simulink model "RealAndSimulatedPlantBlock2019"  (R2019b)
settings: Solver=FixedStepAuto  StartTime=0.0  StopTime=60  FixedStep=0.001  RelTol=1e-3
values from neighbouring files (symbols this model uses):
  A = [0 0 0 0 1 -7.46314951586 0 9.2203186001 0 -3.6743536316 0 36.5167723042 ... (16 elements, 4x4)]    [PlantParams.mat]
  B = [0 5.59662878796 0 -6.91433293703]    [PlantParams.mat]
  c = 0.2    [PlantParams.mat]    (also in params.m = 0.1)
  dtheta1 = 41.8879020479    [PlantParams.mat]    (also in params.m)
  g = 9.81    [PlantParams.mat]    (also in params.m)
  Id = 0.0148    [PlantParams.mat]    (also in params.m)
  ID = 0.0148142940058    [PlantParams.mat]
  J1 = 0.13138281053    [PlantParams.mat]    (also in params.m = 0.1314)
  JC = 0.0268600431258    [PlantParams.mat]
  JD = 0.0273039035837    [PlantParams.mat]
  Jz_bar = 0.0130765    [PlantParams.mat]    (also in params.m = 0.0131)
  lcg = 0.269778481013    [PlantParams.mat]    (also in params.m = 0.2698)
  m = 0.158    [PlantParams.mat]    (also in params.m)
  rh = 0.37    [PlantParams.mat]    (also in params.m)
undefined symbols (not defined in the file or in its folder): C, D, X, Y, Z
libraries: sm_lib x20, nesl_utility x5, simulink x1
(part 1 of 2)
settings Model: EnablePacing=on  Creator=samue  LastModifiedBy=samue
settings DebuggingCC: SFMachineParentedDataDiag=error

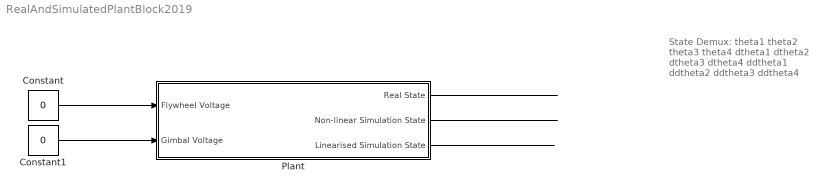
== system RealAndSimulatedPlantBlock2019 ==
  note: State Demux:
      | theta1
      | theta2
      | theta3
      | theta4
      | dtheta1
      | dtheta2
      | dtheta3
      | dtheta4
      | ddtheta1
      | ddtheta2
      | ddtheta3
      | ddtheta4
  Constant : Constant  Value=0
  Constant1 : Constant  Value=0
  Plant : Subsystem
  wires:
  Constant/1 -> Plant/1(Flywheel Voltage)
  Constant1/1 -> Plant/2(Gimbal Voltage)
  Plant/1(Real State) -> ?
  Plant/2(Non-linear Simulation State) -> ?
  Plant/3(Linearised Simulation State) -> ?

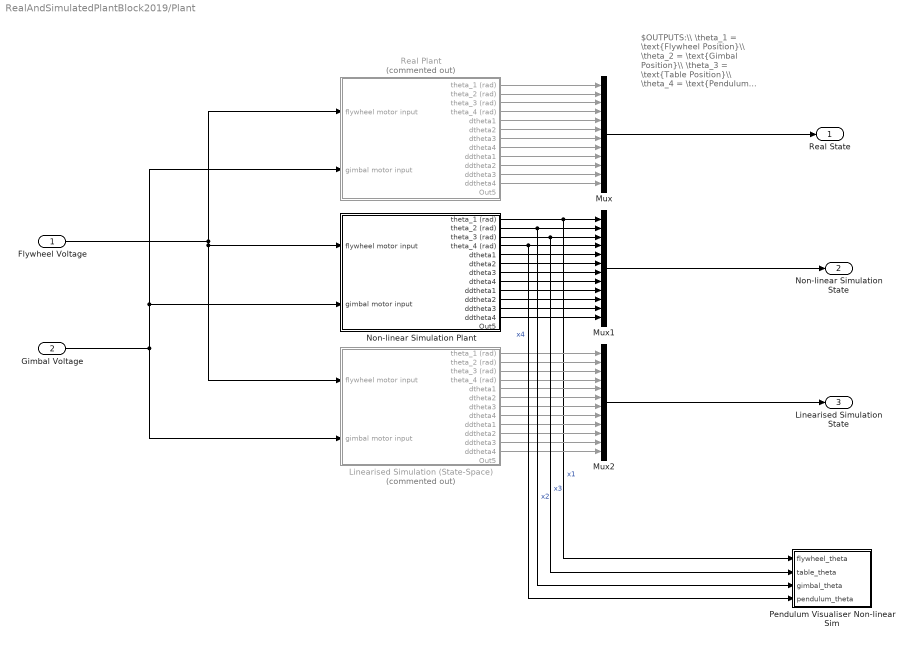
== system RealAndSimulatedPlantBlock2019/Plant ==
  note: $OUTPUTS:\\ \theta_1 = \text{Flywheel Position}\\ \theta_2 = \text{Gimbal Position}\\ \theta_3 = \text{Table Position}\\ \theta_4 = \text{Pendulum Position}\\$
  Flywheel Voltage : Inport
  Gimbal Voltage : Inport  Port=2
  Linearised Simulation (State-Space) : Subsystem  Commented=on
  Mux : Mux  Inputs=12
  Mux1 : Mux  Inputs=12
  Mux2 : Mux  Inputs=12
  Non-linear Simulation Plant : Subsystem
  Pendulum Visualiser Non-linear Sim : Subsystem
  Real Plant : Subsystem  Commented=on
  Real State : Outport
  Non-linear Simulation State : Outport  Port=2
  Linearised Simulation State : Outport  Port=3
  wires:
  Gimbal Voltage/1 -> Linearised Simulation (State-Space)/2(gimbal motor input), Real Plant/2(gimbal motor input), Non-linear Simulation Plant/2(gimbal motor input)
  Flywheel Voltage/1 -> Linearised Simulation (State-Space)/1(flywheel motor input), Non-linear Simulation Plant/1(flywheel motor input), Real Plant/1(flywheel motor input)
  Real Plant/3(theta_3 (rad)) -> Mux/3
  Real Plant/1(theta_1 (rad)) -> Mux/1
  Real Plant/4(theta_4 (rad)) -> Mux/4
  Real Plant/2(theta_2 (rad)) -> Mux/2
  Real Plant/5(dtheta1) -> Mux/5
  Real Plant/6(dtheta2) -> Mux/6
  Real Plant/7(dtheta3) -> Mux/7
  Real Plant/8(dtheta4) -> Mux/8
  Real Plant/9(ddtheta1) -> Mux/9
  Real Plant/10(ddtheta2) -> Mux/10
  Real Plant/11(ddtheta3) -> Mux/11
  Real Plant/12(ddtheta4) -> Mux/12
  Mux/1 -> Real State/1
  Non-linear Simulation Plant/9(ddtheta1) -> Mux1/9
  Non-linear Simulation Plant/12(ddtheta4) -> Mux1/12
  Non-linear Simulation Plant/1(theta_1 (rad)) -> Pendulum Visualiser Non-linear Sim/1(flywheel_theta), Mux1/1  "x1"
  Non-linear Simulation Plant/7(dtheta3) -> Mux1/7
  Non-linear Simulation Plant/10(ddtheta2) -> Mux1/10
  Non-linear Simulation Plant/11(ddtheta3) -> Mux1/11
  Non-linear Simulation Plant/8(dtheta4) -> Mux1/8
  Non-linear Simulation Plant/6(dtheta2) -> Mux1/6
  Non-linear Simulation Plant/5(dtheta1) -> Mux1/5
  Mux1/1 -> Non-linear Simulation State/1
  Linearised Simulation (State-Space)/3(theta_3 (rad)) -> Mux2/3
  Linearised Simulation (State-Space)/9(ddtheta1) -> Mux2/9
  Linearised Simulation (State-Space)/4(theta_4 (rad)) -> Mux2/4
  Linearised Simulation (State-Space)/7(dtheta3) -> Mux2/7
  Linearised Simulation (State-Space)/5(dtheta1) -> Mux2/5
  Linearised Simulation (State-Space)/12(ddtheta4) -> Mux2/12
  Linearised Simulation (State-Space)/1(theta_1 (rad)) -> Mux2/1
  Linearised Simulation (State-Space)/10(ddtheta2) -> Mux2/10
  Linearised Simulation (State-Space)/11(ddtheta3) -> Mux2/11
  Linearised Simulation (State-Space)/8(dtheta4) -> Mux2/8
  Mux2/1 -> Linearised Simulation State/1
  Linearised Simulation (State-Space)/6(dtheta2) -> Mux2/6
  Linearised Simulation (State-Space)/2(theta_2 (rad)) -> Mux2/2
  Non-linear Simulation Plant/4(theta_4 (rad)) -> Pendulum Visualiser Non-linear Sim/4(pendulum_theta), Mux1/4  "x4"
  Non-linear Simulation Plant/2(theta_2 (rad)) -> Pendulum Visualiser Non-linear Sim/3(gimbal_theta), Mux1/2  "x2"
  Non-linear Simulation Plant/3(theta_3 (rad)) -> Pendulum Visualiser Non-linear Sim/2(table_theta), Mux1/3  "x3"

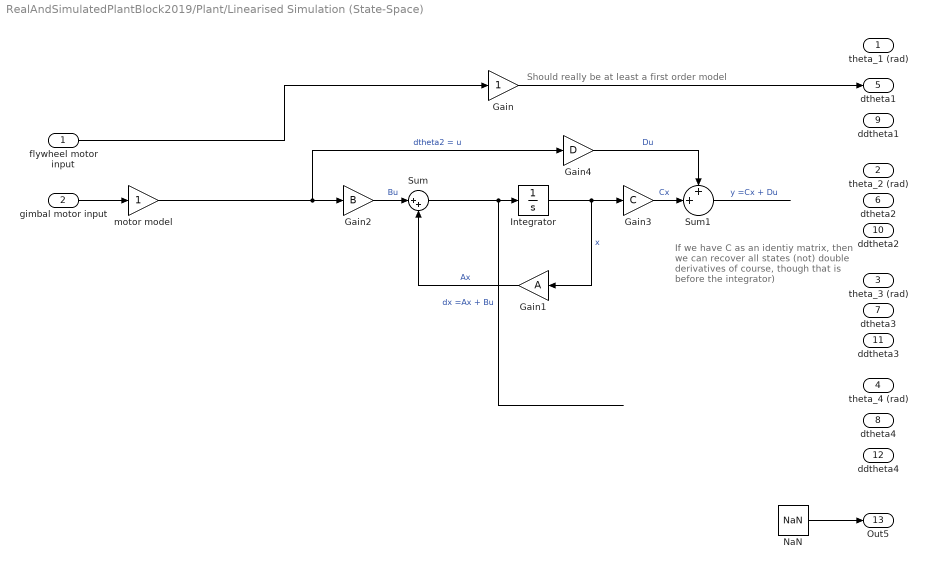
== system RealAndSimulatedPlantBlock2019/Plant/Linearised Simulation (State-Space) ==
  note: If we have C as an identiy matrix,
      | then we can recover all states (not)
      | double derivatives of course, though
      | that is before the integrator)
  note: Should really be at least a first order model
  flywheel motor input : Inport
  gimbal motor input : Inport  Port=2
  Gain : Gain
  Gain1 : Gain  Gain=A
  Gain2 : Gain  Gain=B
  Gain3 : Gain  Gain=C
  Gain4 : Gain  Gain=D
  Integrator : Integrator
  NaN : Constant  Value=NaN  OutDataTypeStr=Inherit: Inherit via back propagation
  Sum : Sum  Inputs=|++
  Sum1 : Sum  Inputs=++|
  motor model : Gain
  theta_1 (rad) : Outport
  theta_2 (rad) : Outport  Port=2
  theta_3 (rad) : Outport  Port=3
  theta_4 (rad) : Outport  Port=4
  dtheta1 : Outport  Port=5
  dtheta2 : Outport  Port=6
  dtheta3 : Outport  Port=7
  dtheta4 : Outport  Port=8
  ddtheta1 : Outport  Port=9
  ddtheta2 : Outport  Port=10
  ddtheta3 : Outport  Port=11
  ddtheta4 : Outport  Port=12
  Out5 : Outport  Port=13
  wires:
  gimbal motor input/1 -> motor model/1
  NaN/1 -> Out5/1
  flywheel motor input/1 -> Gain/1
  Gain/1 -> dtheta1/1
  Integrator/1 -> Gain3/1, Gain1/1  "x"
  Gain1/1 -> Sum/2  "Ax"
  Sum/1 -> Integrator/1  "dx =Ax + Bu"
  Gain2/1 -> Sum/1  "Bu"
  motor model/1 -> Gain2/1, Gain4/1  "dtheta2 = u"
  Gain3/1 -> Sum1/2  "Cx"
  Gain4/1 -> Sum1/1  "Du"
  Sum1/1 -> ?  "y =Cx + Du"

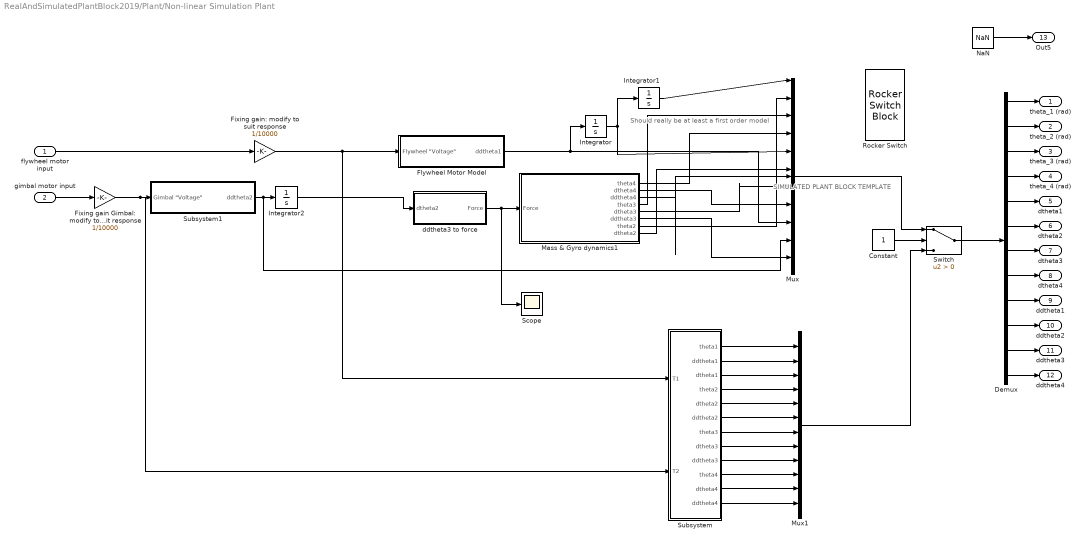
== system RealAndSimulatedPlantBlock2019/Plant/Non-linear Simulation Plant ==
  note: SIMULATED PLANT BLOCK TEMPLATE
  note: Should really be at least a first order model
  flywheel motor input : Inport
  gimbal motor input : Inport  Port=2
  Constant : Constant
  Demux : Demux  Outputs=12
  Fixing gain Gimbal: modify to suit response : Gain  Gain=1/10000
  Fixing gain: modify to suit response : Gain  Gain=1/10000
  "Flywheel Motor Model " : Subsystem
  Integrator : Integrator
  Integrator1 : Integrator
  Integrator2 : Integrator
  Mass & Gyro dynamics1 : Subsystem
  Mux : Mux  Inputs=12
  Mux1 : Mux  Inputs=12
  NaN : Constant  Value=NaN  OutDataTypeStr=Inherit: Inherit via back propagation
  Rocker Switch : RockerSwitchBlock
      settings: Values={{'Off', 'On'}, [0 1]}
  Scope : Scope
  Subsystem : Subsystem
  Subsystem1 : Subsystem
  Switch : Switch  Criteria=u2 > Threshold
  ddtheta3 to force : Subsystem
  theta_1 (rad) : Outport
  theta_2 (rad) : Outport  Port=2
  theta_3 (rad) : Outport  Port=3
  theta_4 (rad) : Outport  Port=4
  dtheta1 : Outport  Port=5
  dtheta2 : Outport  Port=6
  dtheta3 : Outport  Port=7
  dtheta4 : Outport  Port=8
  ddtheta1 : Outport  Port=9
  ddtheta2 : Outport  Port=10
  ddtheta3 : Outport  Port=11
  ddtheta4 : Outport  Port=12
  Out5 : Outport  Port=13
  wires:
  gimbal motor input/1 -> Fixing gain Gimbal: modify to suit response/1
  NaN/1 -> Out5/1
  Subsystem1/1(ddtheta2) -> Mux/10, Integrator2/1
  Mass & Gyro dynamics1/7(theta2) -> Mux/2
  Mass & Gyro dynamics1/8(dtheta2) -> Mux/6
  Mass & Gyro dynamics1/4(theta3) -> Mux/3
  Mass & Gyro dynamics1/5(dtheta3) -> Mux/7
  Mass & Gyro dynamics1/6(ddtheta3) -> Mux/11
  Mass & Gyro dynamics1/1(theta4) -> Mux/4
  Mass & Gyro dynamics1/2(dtheta4) -> Mux/8
  Mass & Gyro dynamics1/3(ddtheta4) -> Mux/12
  flywheel motor input/1 -> Fixing gain: modify to suit response/1
  ddtheta3 to force/1(Force) -> Scope/1, Mass & Gyro dynamics1/1(Force)
  Integrator2/1 -> ddtheta3 to force/1(dtheta2)
  "Flywheel Motor Model "/1(ddtheta1) -> Mux/9, Integrator/1
  Fixing gain: modify to suit response/1 -> Subsystem/1(T1), "Flywheel Motor Model "/1("Flywheel \"Voltage\"")
  Integrator/1 -> Integrator1/1, Mux/5
  Integrator1/1 -> Mux/1
  Fixing gain Gimbal: modify to suit response/1 -> Subsystem/2(T2), Subsystem1/1("Gimbal \"Voltage\"")
  Subsystem/1(theta1) -> Mux1/1
  Subsystem/2(ddtheta1) -> Mux1/2
  Subsystem/3(dtheta1) -> Mux1/3
  Subsystem/4("theta2 ") -> Mux1/4
  Subsystem/6(ddtheta2) -> Mux1/6
  Subsystem/5(dtheta2) -> Mux1/5
  Subsystem/7(theta3) -> Mux1/7
  Subsystem/8(dtheta3) -> Mux1/8
  Subsystem/9(ddtheta3) -> Mux1/9
  Subsystem/10(theta4) -> Mux1/10
  Subsystem/11(dtheta4) -> Mux1/11
  Subsystem/12("ddtheta4 ") -> Mux1/12
  Demux/1 -> theta_1 (rad)/1
  Demux/2 -> theta_2 (rad)/1
  Demux/3 -> theta_3 (rad)/1
  Demux/4 -> theta_4 (rad)/1
  Demux/5 -> dtheta1/1
  Demux/6 -> dtheta2/1
  Demux/7 -> dtheta3/1
  Demux/8 -> dtheta4/1
  Demux/9 -> ddtheta1/1
  Demux/10 -> ddtheta2/1
  Demux/11 -> ddtheta3/1
  Demux/12 -> ddtheta4/1
  Constant/1 -> Switch/2
  Mux/1 -> Switch/1
  Mux1/1 -> Switch/3
  Switch/1 -> Demux/1

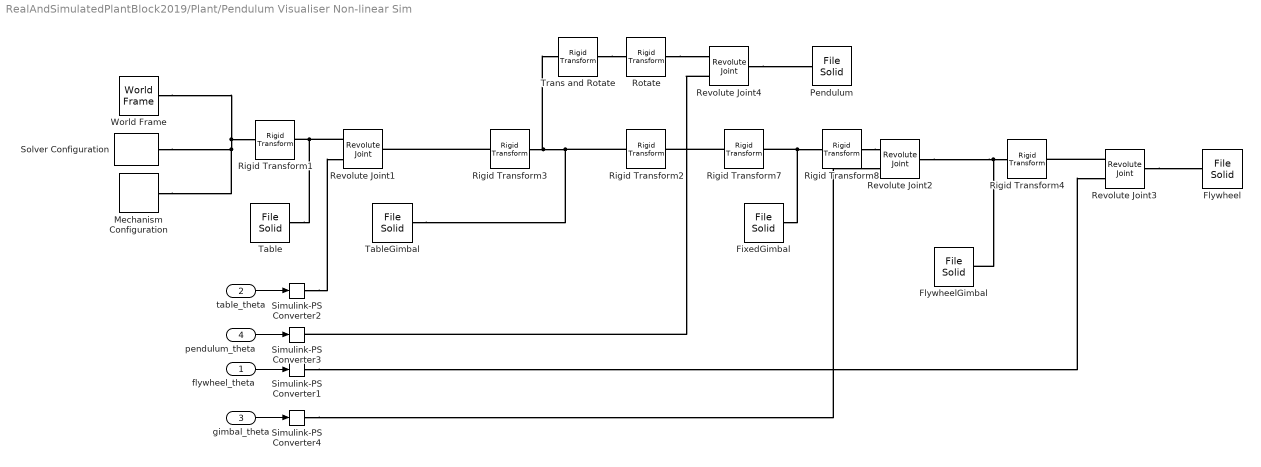
== system RealAndSimulatedPlantBlock2019/Plant/Pendulum Visualiser Non-linear Sim ==
  flywheel_theta : Inport
  table_theta : Inport  Port=2
  gimbal_theta : Inport  Port=3
  pendulum_theta : Inport  Port=4
  FixedGimbal : sm_lib/Body Elements/File Solid  ExtGeomFileName=C:\Users\samue\OneDrive\METR6203\CAD\gimbal_fixed.stp  UnitType=FromFile  ExtGeomFileUnits=m  StepReaderType=HEX  ExportEntireGeometry=off  InertiaType=CalculateFromGeometry  Mass=1  MassUnits=kg  CenterOfMass=[0 0 0]  CenterOfMassUnits=m  MomentsOfInertia=[1 1 1]  MomentsOfInertiaUnits=kg*m^2  ProductsOfInertia=[0 0 0]  ProductsOfInertiaUnits=kg*m^2  BasedOnType=Density  Density=1000  DensityUnits=kg/m^3  DoExposeReferenceFrame=on  SerializedFrames=<Frames/>  GraphicType=FromGeometry  MarkerShape=Sphere  MarkerSize=10  GraphicVisPropType=SimpleVisualProperties  GraphicDiffuseColor=[0.2 0.2 0.2]  GraphicSpecularColor=[0.5 0.5 0.5 1.0]  GraphicAmbientColor=[0.15 0.15 0.15 1.0]  GraphicEmissiveColor=[0.0 0.0 0.0 1.0]  GraphicShininess=75  GraphicOpacity=1.0
  Flywheel : sm_lib/Body Elements/File Solid  ExtGeomFileName=C:\Users\samue\OneDrive\METR6203\CAD\flywheel.stp  UnitType=FromFile  ExtGeomFileUnits=m  StepReaderType=HEX  ExportEntireGeometry=off  InertiaType=CalculateFromGeometry  Mass=1  MassUnits=kg  CenterOfMass=[0 0 0]  CenterOfMassUnits=m  MomentsOfInertia=[1 1 1]  MomentsOfInertiaUnits=kg*m^2  ProductsOfInertia=[0 0 0]  ProductsOfInertiaUnits=kg*m^2  BasedOnType=Density  Density=1000  DensityUnits=kg/m^3  DoExposeReferenceFrame=on  SerializedFrames=<Frames/>  GraphicType=FromGeometry  MarkerShape=Sphere  MarkerSize=10  GraphicVisPropType=SimpleVisualProperties  GraphicDiffuseColor=[0.8 0.6 0.0]  GraphicSpecularColor=[0.5 0.5 0.5 1.0]  GraphicAmbientColor=[0.15 0.15 0.15 1.0]  GraphicEmissiveColor=[0.0 0.0 0.0 1.0]  GraphicShininess=75  GraphicOpacity=1.0
  FlywheelGimbal : sm_lib/Body Elements/File Solid  ExtGeomFileName=C:\Users\samue\OneDrive\METR6203\CAD\flywheel_gimbal.stp  UnitType=FromFile  ExtGeomFileUnits=m  StepReaderType=HEX  ExportEntireGeometry=off  InertiaType=CalculateFromGeometry  Mass=1  MassUnits=kg  CenterOfMass=[0 0 0]  CenterOfMassUnits=m  MomentsOfInertia=[1 1 1]  MomentsOfInertiaUnits=kg*m^2  ProductsOfInertia=[0 0 0]  ProductsOfInertiaUnits=kg*m^2  BasedOnType=Density  Density=1000  DensityUnits=kg/m^3  DoExposeReferenceFrame=on  SerializedFrames=<Frames/>  GraphicType=FromGeometry  MarkerShape=Sphere  MarkerSize=10  GraphicVisPropType=SimpleVisualProperties  GraphicDiffuseColor=[0.5 0.5 0.5]  GraphicSpecularColor=[0.5 0.5 0.5 1.0]  GraphicAmbientColor=[0.15 0.15 0.15 1.0]  GraphicEmissiveColor=[0.0 0.0 0.0 1.0]  GraphicShininess=75  GraphicOpacity=1.0
  Mechanism Configuration : sm_lib/Utilities/Mechanism Configuration  UniformGravity=Constant  GravityVector=[0 0 -9.80665]  GravityUnits=m/s^2  LinearizationDelta=0.001
  Pendulum : sm_lib/Body Elements/File Solid  ExtGeomFileName=C:\Users\samue\OneDrive\METR6203\CAD\pendulum.stp  UnitType=FromFile  ExtGeomFileUnits=m  StepReaderType=HEX  ExportEntireGeometry=off  InertiaType=CalculateFromGeometry  Mass=1  MassUnits=kg  CenterOfMass=[0 0 0]  CenterOfMassUnits=m  MomentsOfInertia=[1 1 1]  MomentsOfInertiaUnits=kg*m^2  ProductsOfInertia=[0 0 0]  ProductsOfInertiaUnits=kg*m^2  BasedOnType=Density  Density=1000  DensityUnits=kg/m^3  DoExposeReferenceFrame=on  SerializedFrames=<Frames/>  GraphicType=FromGeometry  MarkerShape=Sphere  MarkerSize=10  GraphicVisPropType=SimpleVisualProperties  GraphicDiffuseColor=[0.5 0.5 0.5]  GraphicSpecularColor=[0.5 0.5 0.5 1.0]  GraphicAmbientColor=[0.15 0.15 0.15 1.0]  GraphicEmissiveColor=[0.0 0.0 0.0 1.0]  GraphicShininess=75  GraphicOpacity=1.0
  Revolute Joint{1..4} (4 alike) : sm_lib/Joints/Revolute Joint  JointMode=Normal  SenseConstraintForce=off  SenseConstraintForceX=off  SenseConstraintForceY=off  SenseConstraintForceZ=off  SenseConstraintTorque=off  SenseConstraintTorqueX=off  SenseConstraintTorqueY=off  SenseConstraintTorqueZ=off  SenseTotalForce=off  SenseTotalForceX=off  SenseTotalForceY=off  SenseTotalForceZ=off  SenseTotalTorque=off  SenseTotalTorqueX=off  SenseTotalTorqueY=off  SenseTotalTorqueZ=off  CompositeWrenchDir=FollowerOnBase  CompositeWrenchFrame=BaseFrame  EquilibriumPosition=0  EquilibriumPositionUnits=deg  SpringStiffness=0  SpringStiffnessUnits=N*m/deg  DampingCoefficient=0  DampingCoefficientUnits=N*m/(deg/s)  TorqueActuationMode=ComputedTorque  MotionActuationMode=InputMotion  SensePosition=off  SenseVelocity=off  SenseAcceleration=off  SenseTorqueForce=off  SenseLowerLimitTorqueForce=off  SenseUpperLimitTorqueForce=off  LowerLimitSpecify=off  LowerLimitBound=-90  LowerLimitBoundUnits=deg  LowerLimitStiffness=1e4  LowerLimitStiffnessUnits=N*m/deg  LowerLimitDamping=10  LowerLimitDampingUnits=N*m/(deg/s)  LowerLimitTransitionRegionWidth=0.1  LowerLimitTransitionRegionWidthUnits=deg  UpperLimitSpecify=off  UpperLimitBound=90  UpperLimitBoundUnits=deg  UpperLimitStiffness=1e4  UpperLimitStiffnessUnits=N*m/deg  UpperLimitDamping=10  UpperLimitDampingUnits=N*m/(deg/s)  UpperLimitTransitionRegionWidth=0.1  UpperLimitTransitionRegionWidthUnits=deg  PositionTargetSpecify=off  PositionTargetPriority=High  PositionTargetValue=0  PositionTargetValueUnits=deg  VelocityTargetSpecify=off  VelocityTargetPriority=High  VelocityTargetValue=0  VelocityTargetValueUnits=deg/s
  Rigid Transform1 : sm_lib/Frames and Transforms/Rigid Transform  TranslationMethod=None  TranslationStandardOffset=0  TranslationLengthUnit=m  TranslationStandardAxis=+Z  TranslationCartesianOffset=[0 0 0]  TranslationROffset=0  TranslationROffsetUnits=m  TranslationZOffset=0  TranslationZOffsetUnits=m  TranslationThetaOffset=0  TranslationThetaOffsetUnits=deg  RotationMethod=StandardAxis  RotationAngleUnits=deg  RotationStandardAxis=+X  RotationAngle=0  RotationArbitraryAxis=[0 0 1]  FollAlignAxisA=+X  BaseAlignAxisA=+Y  FollAlignAxisB=+Y  BaseAlignAxisB=+Z  RotationSequenceAxes=FollowerAxes  RotationSequence=XYX  RotationSequenceAngles=[0 0 0]  RotationSequenceAnglesUnits=deg  RotationMatrix=[1 0 0; 0 1 0; 0 0 1]
  Rigid Transform2 : sm_lib/Frames and Transforms/Rigid Transform  TranslationMethod=StandardAxis  TranslationStandardOffset=00  TranslationLengthUnit=m  TranslationStandardAxis=+Y  TranslationCartesianOffset=[0 0 0]  TranslationROffset=0  TranslationROffsetUnits=m  TranslationZOffset=0  TranslationZOffsetUnits=m  TranslationThetaOffset=0  TranslationThetaOffsetUnits=deg  RotationMethod=StandardAxis  RotationAngleUnits=deg  RotationStandardAxis=+X  RotationAngle=90  RotationArbitraryAxis=[0 0 1]  FollAlignAxisA=+X  BaseAlignAxisA=+Y  FollAlignAxisB=+Y  BaseAlignAxisB=+Z  RotationSequenceAxes=FollowerAxes  RotationSequence=XYX  RotationSequenceAngles=[0 0 0]  RotationSequenceAnglesUnits=deg  RotationMatrix=[1 0 0; 0 1 0; 0 0 1]
  Rigid Transform3 : sm_lib/Frames and Transforms/Rigid Transform  TranslationMethod=StandardAxis  TranslationStandardOffset=245+7  TranslationLengthUnit=mm  TranslationStandardAxis=+Z  TranslationCartesianOffset=[0 0 0]  TranslationROffset=0  TranslationROffsetUnits=m  TranslationZOffset=0  TranslationZOffsetUnits=m  TranslationThetaOffset=0  TranslationThetaOffsetUnits=deg  RotationMethod=StandardAxis  RotationAngleUnits=deg  RotationStandardAxis=+X  RotationAngle=0  RotationArbitraryAxis=[0 0 1]  FollAlignAxisA=+X  BaseAlignAxisA=+Y  FollAlignAxisB=+Y  BaseAlignAxisB=+Z  RotationSequenceAxes=FollowerAxes  RotationSequence=XYX  RotationSequenceAngles=[0 0 0]  RotationSequenceAnglesUnits=deg  RotationMatrix=[1 0 0; 0 1 0; 0 0 1]
  Rigid Transform4 : sm_lib/Frames and Transforms/Rigid Transform  TranslationMethod=StandardAxis  TranslationStandardOffset=00  TranslationLengthUnit=m  TranslationStandardAxis=+Y  TranslationCartesianOffset=[0 0 0]  TranslationROffset=0  TranslationROffsetUnits=m  TranslationZOffset=0  TranslationZOffsetUnits=m  TranslationThetaOffset=0  TranslationThetaOffsetUnits=deg  RotationMethod=StandardAxis  RotationAngleUnits=deg  RotationStandardAxis=+Y  RotationAngle=90  RotationArbitraryAxis=[0 0 1]  FollAlignAxisA=+X  BaseAlignAxisA=+Y  FollAlignAxisB=+Y  BaseAlignAxisB=+Z  RotationSequenceAxes=FollowerAxes  RotationSequence=XYX  RotationSequenceAngles=[0 0 0]  RotationSequenceAnglesUnits=deg  RotationMatrix=[1 0 0; 0 1 0; 0 0 1]
  Rigid Transform7 : sm_lib/Frames and Transforms/Rigid Transform  TranslationMethod=StandardAxis  TranslationStandardOffset=00  TranslationLengthUnit=m  TranslationStandardAxis=+Y  TranslationCartesianOffset=[0 0 0]  TranslationROffset=0  TranslationROffsetUnits=m  TranslationZOffset=0  TranslationZOffsetUnits=m  TranslationThetaOffset=0  TranslationThetaOffsetUnits=deg  RotationMethod=StandardAxis  RotationAngleUnits=deg  RotationStandardAxis=+Y  RotationAngle=90  RotationArbitraryAxis=[0 0 1]  FollAlignAxisA=+X  BaseAlignAxisA=+Y  FollAlignAxisB=+Y  BaseAlignAxisB=+Z  RotationSequenceAxes=FollowerAxes  RotationSequence=XYX  RotationSequenceAngles=[0 0 0]  RotationSequenceAnglesUnits=deg  RotationMatrix=[1 0 0; 0 1 0; 0 0 1]
  Rigid Transform8 : sm_lib/Frames and Transforms/Rigid Transform  TranslationMethod=StandardAxis  TranslationStandardOffset=00  TranslationLengthUnit=m  TranslationStandardAxis=+Y  TranslationCartesianOffset=[0 0 0]  TranslationROffset=0  TranslationROffsetUnits=m  TranslationZOffset=0  TranslationZOffsetUnits=m  TranslationThetaOffset=0  TranslationThetaOffsetUnits=deg  RotationMethod=StandardAxis  RotationAngleUnits=deg  RotationStandardAxis=-Y  RotationAngle=90  RotationArbitraryAxis=[0 0 1]  FollAlignAxisA=+X  BaseAlignAxisA=+Y  FollAlignAxisB=+Y  BaseAlignAxisB=+Z  RotationSequenceAxes=FollowerAxes  RotationSequence=XYX  RotationSequenceAngles=[0 0 0]  RotationSequenceAnglesUnits=deg  RotationMatrix=[1 0 0; 0 1 0; 0 0 1]
  Rotate : sm_lib/Frames and Transforms/Rigid Transform  TranslationMethod=StandardAxis  TranslationStandardOffset=320-245  TranslationLengthUnit=mm  TranslationStandardAxis=-X  TranslationCartesianOffset=[0 0 0]  TranslationROffset=0  TranslationROffsetUnits=m  TranslationZOffset=0  TranslationZOffsetUnits=m  TranslationThetaOffset=0  TranslationThetaOffsetUnits=deg  RotationMethod=StandardAxis  RotationAngleUnits=deg  RotationStandardAxis=+Z  RotationAngle=90  RotationArbitraryAxis=[0 0 1]  FollAlignAxisA=+X  BaseAlignAxisA=+Y  FollAlignAxisB=+Y  BaseAlignAxisB=+Z  RotationSequenceAxes=FollowerAxes  RotationSequence=XYX  RotationSequenceAngles=[0 0 0]  RotationSequenceAnglesUnits=deg  RotationMatrix=[1 0 0; 0 1 0; 0 0 1]
  Simulink-PS Converter{1..4} (4 alike) : nesl_utility/Simulink-PS Converter  PhysicalDomain=network_engine_domain  SubClassName=ps_input  LeftPortType=input  RightPortType=output  PseudoPeriodic=off  Frequencies=[]  NoiseDistribution=none  NoiseParameters=[]  Unit=rad  AffineConversion=off  FilteringAndDerivatives=filter  SimscapeFilterOrder=2  InputFilterTimeConstant=0.001  UdotUserProvided=0
      settings: SourceProductBaseCode=PW,SS
  Solver Configuration : nesl_utility/Solver Configuration  PhysicalDomain=network_engine_domain  SubClassName=solver  LeftPortType=input  RightPortType=generic  Tones=[]  Harmonics=[]  SimulateNoise=off  Profile=off  UseLocalSampling=off  EnableSwitchedLinearOptims=on  FrequencyDomain=off  UseCCode=off  RelTol=0.001  AbsTol=1e-06  MinStep=1e-09  ToWorkspace=off  RevertToSquareIcSolve=off  NumHomotopyIterations=100  PhasorMode=off  PhasorModeNumHarmonics=1  DoDC=off  ResidualTolerance=1e-09  UseLocalSolver=off  LocalSolverChoice=NE_BACKWARD_EULER_ADVANCER  LocalSolverSampleTime=0.001  DoFixedCost=off  MaxNonlinIter=3  MaxModeIter=2  LinearAlgebra=Full  EquationFormulation=NE_TIME_EF  DelaysMemoryBudget=1024  AutomaticFiltering=on  FilteringTimeConstant=0.001  PartitionStorageMethod=AS_NEEDED  PartitionMemoryBudget=1024  PartitionMethod=ROBUST
      settings: SourceProductBaseCode=PW,SS
  Table : sm_lib/Body Elements/File Solid  ExtGeomFileName=C:\Users\samue\OneDrive\METR6203\CAD\base_link.stp  UnitType=FromFile  ExtGeomFileUnits=m  StepReaderType=HEX  ExportEntireGeometry=off  InertiaType=CalculateFromGeometry  Mass=1  MassUnits=kg  CenterOfMass=[0 0 0]  CenterOfMassUnits=m  MomentsOfInertia=[1 1 1]  MomentsOfInertiaUnits=kg*m^2  ProductsOfInertia=[0 0 0]  ProductsOfInertiaUnits=kg*m^2  BasedOnType=Density  Density=1000  DensityUnits=kg/m^3  DoExposeReferenceFrame=on  SerializedFrames=<Frames/>  GraphicType=FromGeometry  MarkerShape=Sphere  MarkerSize=10  GraphicVisPropType=SimpleVisualProperties  GraphicDiffuseColor=[0.5 0.5 0.5]  GraphicSpecularColor=[0.5 0.5 0.5 1.0]  GraphicAmbientColor=[0.15 0.15 0.15 1.0]  GraphicEmissiveColor=[0.0 0.0 0.0 1.0]  GraphicShininess=75  GraphicOpacity=1.0
  TableGimbal : sm_lib/Body Elements/File Solid  ExtGeomFileName=C:\Users\samue\OneDrive\METR6203\CAD\gimbal_table.stp  UnitType=FromFile  ExtGeomFileUnits=m  StepReaderType=HEX  ExportEntireGeometry=off  InertiaType=CalculateFromGeometry  Mass=1  MassUnits=kg  CenterOfMass=[0 0 0]  CenterOfMassUnits=m  MomentsOfInertia=[1 1 1]  MomentsOfInertiaUnits=kg*m^2  ProductsOfInertia=[0 0 0]  ProductsOfInertiaUnits=kg*m^2  BasedOnType=Density  Density=1000  DensityUnits=kg/m^3  DoExposeReferenceFrame=on  SerializedFrames=<Frames/>  GraphicType=FromGeometry  MarkerShape=Sphere  MarkerSize=10  GraphicVisPropType=SimpleVisualProperties  GraphicDiffuseColor=[0.5 0.5 0.5]  GraphicSpecularColor=[0.5 0.5 0.5 1.0]  GraphicAmbientColor=[0.15 0.15 0.15 1.0]  GraphicEmissiveColor=[0.0 0.0 0.0 1.0]  GraphicShininess=75  GraphicOpacity=1.0
  Trans and Rotate : sm_lib/Frames and Transforms/Rigid Transform  TranslationMethod=StandardAxis  TranslationStandardOffset=370  TranslationLengthUnit=mm  TranslationStandardAxis=-X  TranslationCartesianOffset=[0 0 0]  TranslationROffset=0  TranslationROffsetUnits=m  TranslationZOffset=0  TranslationZOffsetUnits=m  TranslationThetaOffset=0  TranslationThetaOffsetUnits=deg  RotationMethod=StandardAxis  RotationAngleUnits=deg  RotationStandardAxis=+Y  RotationAngle=90  RotationArbitraryAxis=[0 0 1]  FollAlignAxisA=+X  BaseAlignAxisA=+Y  FollAlignAxisB=+Y  BaseAlignAxisB=+Z  RotationSequenceAxes=FollowerAxes  RotationSequence=XYX  RotationSequenceAngles=[0 0 0]  RotationSequenceAnglesUnits=deg  RotationMatrix=[1 0 0; 0 1 0; 0 0 1]
  World Frame : sm_lib/Frames and Transforms/World Frame
  wires:
  flywheel_theta/1 -> Simulink-PS Converter1/1
  table_theta/1 -> Simulink-PS Converter2/1
  pendulum_theta/1 -> Simulink-PS Converter3/1
  gimbal_theta/1 -> Simulink-PS Converter4/1
  connections:
  Rigid Transform3/LConn1 -- Revolute Joint1/RConn1
  Rigid Transform3/RConn1 -- Rigid Transform2/LConn1 -- TableGimbal/RConn1 -- Trans and Rotate/LConn1
  Simulink-PS Converter1/RConn1 -- Revolute Joint3/LConn2
  World Frame/RConn1 -- Mechanism Configuration/RConn1 -- Solver Configuration/RConn1 -- Rigid Transform1/LConn1
  Simulink-PS Converter2/RConn1 -- Revolute Joint1/LConn2
  Revolute Joint1/LConn1 -- Table/RConn1 -- Rigid Transform1/RConn1
  FixedGimbal/RConn1 -- Rigid Transform8/LConn1 -- Rigid Transform7/RConn1
  Rigid Transform4/LConn1 -- Revolute Joint2/RConn1 -- FlywheelGimbal/RConn1
  Revolute Joint3/LConn1 -- Rigid Transform4/RConn1
  Revolute Joint3/RConn1 -- Flywheel/RConn1
  Simulink-PS Converter4/RConn1 -- Revolute Joint2/LConn2
  Revolute Joint4/LConn2 -- Simulink-PS Converter3/RConn1
  Revolute Joint4/RConn1 -- Pendulum/RConn1
  Trans and Rotate/RConn1 -- Rotate/LConn1
  Rotate/RConn1 -- Revolute Joint4/LConn1
  Rigid Transform7/LConn1 -- Rigid Transform2/RConn1
  Rigid Transform8/RConn1 -- Revolute Joint2/LConn1

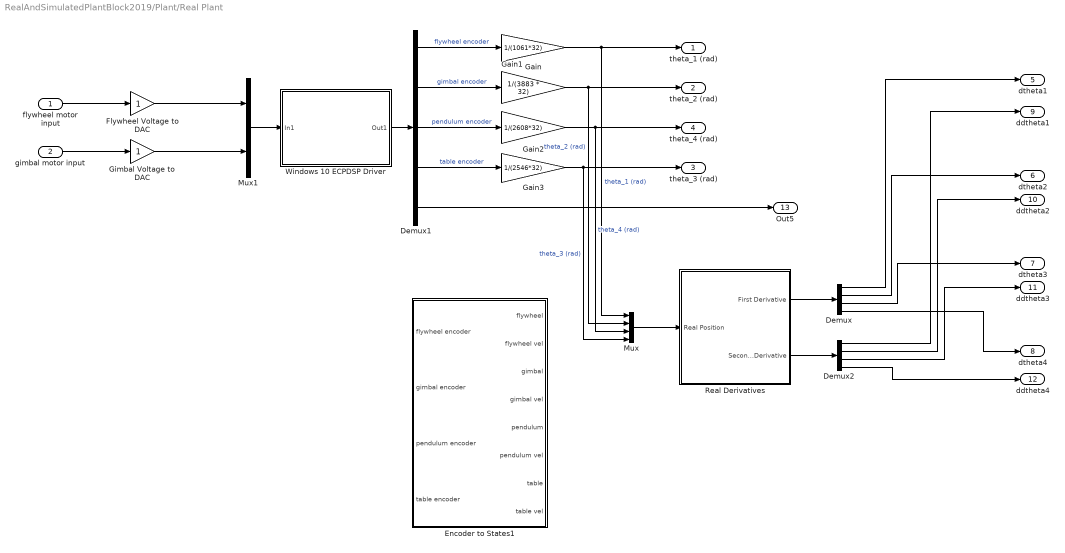
== system RealAndSimulatedPlantBlock2019/Plant/Real Plant ==
  flywheel motor input : Inport
  gimbal motor input : Inport  Port=2
  Demux : Demux
  Demux1 : Demux  Outputs=5
  Demux2 : Demux
  Encoder to States1 : Subsystem
  Flywheel Voltage to DAC : Gain
  Gain : Gain  Gain=1/(1061*32)
  Gain1 : Gain  Gain=1/(3883 * 32)
  Gain2 : Gain  Gain=1/(2608*32)
  Gain3 : Gain  Gain=1/(2546*32)
  Gimbal Voltage to DAC : Gain
  Mux : Mux
  Mux1 : Mux  Inputs=2
  Real Derivatives : Subsystem
  Windows 10 ECPDSP Driver : Subsystem  mask{BaseAddr='0x3F00', STime=0.008, TimeOutPer=500, HWAccess=on}
      mask prompts: BaseAddr "Base I/O Address"; STime "Sample Time (Sec)"; TimeOutPer "Timeout Period (500 ~ 2000)"; HWAccess "Hardware Access"
      mask Display: color('black');disp('ECPDSP Driver\n upto\n 4 Encs(ADC Channels)\n and 2 Dacs')
  theta_1 (rad) : Outport
  theta_2 (rad) : Outport  Port=2
  theta_3 (rad) : Outport  Port=3
  theta_4 (rad) : Outport  Port=4
  dtheta1 : Outport  Port=5
  dtheta2 : Outport  Port=6
  dtheta3 : Outport  Port=7
  dtheta4 : Outport  Port=8
  ddtheta1 : Outport  Port=9
  ddtheta2 : Outport  Port=10
  ddtheta3 : Outport  Port=11
  ddtheta4 : Outport  Port=12
  Out5 : Outport  Port=13
  wires:
  Demux1/2 -> Gain1/1  "gimbal encoder"
  Demux1/1 -> Gain/1  "flywheel encoder"
  Demux1/3 -> Gain2/1  "pendulum encoder"
  Mux1/1 -> Windows 10 ECPDSP Driver/1(In1)
  Demux1/5 -> Out5/1
  Gain1/1 -> Mux/2, theta_2 (rad)/1  "theta_2 (rad)"
  gimbal motor input/1 -> Gimbal Voltage to DAC/1
  Demux1/4 -> Gain3/1  "table encoder"
  Windows 10 ECPDSP Driver/1(Out1) -> Demux1/1
  Gain/1 -> Mux/1, theta_1 (rad)/1  "theta_1 (rad)"
  flywheel motor input/1 -> Flywheel Voltage to DAC/1
  Gain3/1 -> Mux/4, theta_3 (rad)/1  "theta_3 (rad)"
  Gain2/1 -> Mux/3, theta_4 (rad)/1  "theta_4 (rad)"
  Flywheel Voltage to DAC/1 -> Mux1/1
  Gimbal Voltage to DAC/1 -> Mux1/2
  Real Derivatives/2(Second Derivative) -> Demux2/1
  Demux2/1 -> ddtheta1/1
  Demux2/2 -> ddtheta2/1
  Demux2/3 -> ddtheta3/1
  Demux2/4 -> ddtheta4/1
  Real Derivatives/1(First Derivative) -> Demux/1
  Demux/1 -> dtheta1/1
  Demux/2 -> dtheta2/1
  Demux/3 -> dtheta3/1
  Demux/4 -> dtheta4/1
  Mux/1 -> Real Derivatives/1(Real Position)

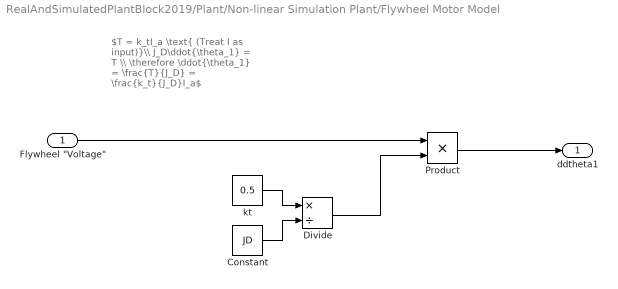
== system RealAndSimulatedPlantBlock2019/Plant/Non-linear Simulation Plant/Flywheel Motor Model  ==
  note: $T = k_tI_a \text{ (Treat I as input)}\\ J_D\ddot{\theta_1} = T \\ \therefore \ddot{\theta_1} = \frac{T}{J_D} = \frac{k_t}{J_D}I_a$
  "Flywheel \"Voltage\"" : Inport
  Constant : Constant  Value=JD
  Divide : Product  Inputs=*/
  Product : Product
  kt : Constant  Value=0.5
  ddtheta1 : Outport
  wires:
  "Flywheel \"Voltage\""/1 -> Product/1
  kt/1 -> Divide/1
  Constant/1 -> Divide/2
  Product/1 -> ddtheta1/1
  Divide/1 -> Product/2

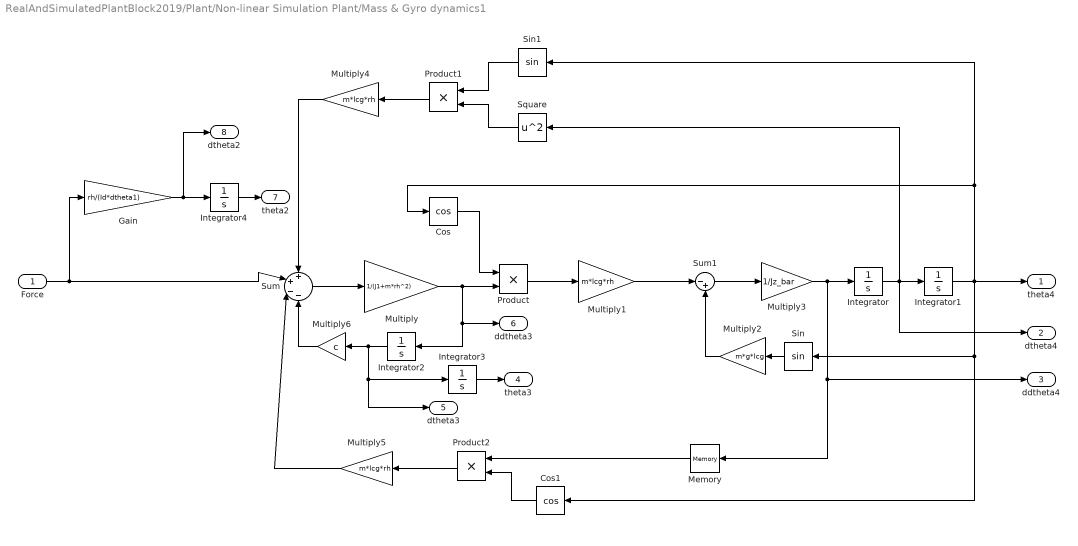
== system RealAndSimulatedPlantBlock2019/Plant/Non-linear Simulation Plant/Mass & Gyro dynamics1 ==
  Force : Inport
  Cos : Trigonometry  Operator=cos
  Cos1 : Trigonometry  Operator=cos
  Gain : Gain  Gain=rh/(Id*dtheta1)
  Integrator{,2..4} (4 alike) : Integrator
  Integrator1 : Integrator  InitialCondition=pi/2
  Memory : Memory
  Multiply : Gain  Gain=1/(J1+m*rh^2)
  Multiply1 : Gain  Gain=m*lcg*rh
  Multiply2 : Gain  Gain=m*g*lcg
  Multiply3 : Gain  Gain=1/Jz_bar
  Multiply4 : Gain  Gain=m*lcg*rh
  Multiply5 : Gain  Gain=m*lcg*rh
  Multiply6 : Gain  Gain=c
  Product : Product
  Product1 : Product
  Product2 : Product
  Sin : Trigonometry
  Sin1 : Trigonometry
  Square : Math  Operator=square  SignedPower=off  SaturateOnIntegerOverflow=on
  Sum : Sum  Inputs=++--
  Sum1 : Sum  Inputs=|-+
  theta4 : Outport
  dtheta4 : Outport  Port=2
  ddtheta4 : Outport  Port=3
  theta3 : Outport  Port=4
  dtheta3 : Outport  Port=5
  ddtheta3 : Outport  Port=6
  theta2 : Outport  Port=7
  dtheta2 : Outport  Port=8
  wires:
  Force/1 -> Sum/2, Gain/1
  Sum/1 -> Multiply/1
  Multiply/1 -> Integrator2/1, ddtheta3/1, Product/2
  Cos/1 -> Product/1
  Product/1 -> Multiply1/1
  Multiply1/1 -> Sum1/1
  Sin/1 -> Multiply2/1
  Multiply2/1 -> Sum1/2
  Sum1/1 -> Multiply3/1
  Multiply3/1 -> ddtheta4/1, Memory/1, Integrator/1
  Integrator/1 -> dtheta4/1, Square/1, Integrator1/1
  Integrator1/1 -> Cos1/1, Sin/1, theta4/1, Cos/1, Sin1/1
  Product1/1 -> Multiply4/1
  Multiply4/1 -> Sum/1
  Sin1/1 -> Product1/1
  Square/1 -> Product1/2
  Product2/1 -> Multiply5/1
  Multiply5/1 -> Sum/3
  Cos1/1 -> Product2/2
  Integrator2/1 -> Multiply6/1, dtheta3/1, Integrator3/1
  Multiply6/1 -> Sum/4
  Integrator3/1 -> theta3/1
  Gain/1 -> dtheta2/1, Integrator4/1
  Integrator4/1 -> theta2/1
  Memory/1 -> Product2/1

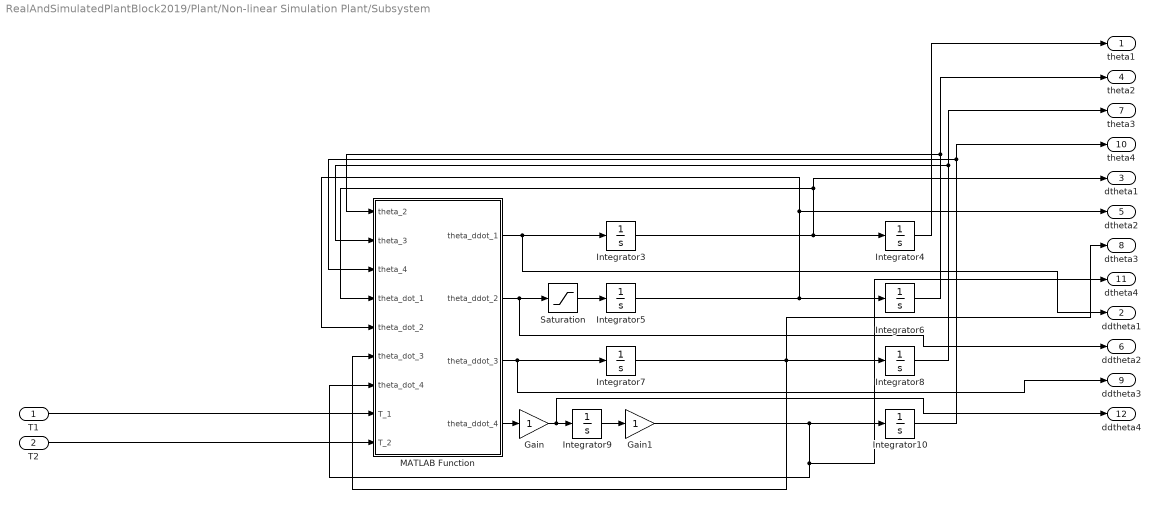
== system RealAndSimulatedPlantBlock2019/Plant/Non-linear Simulation Plant/Subsystem ==
  T1 : Inport
  T2 : Inport  Port=2
  Gain : Gain
  Gain1 : Gain
  Integrator10 : Integrator  InitialCondition=pi
  Integrator3 : Integrator  InitialCondition=400*2*pi/60  LimitOutput=on
  Integrator4 : Integrator
  Integrator5 : Integrator  LimitOutput=on  UpperSaturationLimit=100  LowerSaturationLimit=-100
  Integrator6 : Integrator
  Integrator7 : Integrator  LimitOutput=on  UpperSaturationLimit=100  LowerSaturationLimit=-100
  Integrator8 : Integrator
  Integrator9 : Integrator  InitialCondition=1  LimitOutput=on  UpperSaturationLimit=100  LowerSaturationLimit=-100
  MATLAB Function : MATLAB Function  TreatAsAtomicUnit=on
  Saturation : Saturate  UpperLimit=20  LowerLimit=-20
  theta1 : Outport
  ddtheta1 : Outport  Port=2
  dtheta1 : Outport  Port=3
  "theta2 " : Outport  Port=4
  dtheta2 : Outport  Port=5
  ddtheta2 : Outport  Port=6
  theta3 : Outport  Port=7
  dtheta3 : Outport  Port=8
  ddtheta3 : Outport  Port=9
  theta4 : Outport  Port=10
  dtheta4 : Outport  Port=11
  "ddtheta4 " : Outport  Port=12
  wires:
  Integrator10/1 -> theta4/1, MATLAB Function/3(theta_4)
  MATLAB Function/2(theta_ddot_2) -> ddtheta2/1, Saturation/1
  Integrator6/1 -> "theta2 "/1, MATLAB Function/1(theta_2)
  Integrator9/1 -> Gain1/1
  Gain/1 -> "ddtheta4 "/1, Integrator9/1
  Integrator7/1 -> dtheta3/1, MATLAB Function/6(theta_dot_3), Integrator8/1
  Integrator3/1 -> Integrator4/1, dtheta1/1, MATLAB Function/4(theta_dot_1)
  Integrator4/1 -> theta1/1
  MATLAB Function/1(theta_ddot_1) -> ddtheta1/1, Integrator3/1
  Integrator5/1 -> dtheta2/1, MATLAB Function/5(theta_dot_2), Integrator6/1
  Gain1/1 -> Integrator10/1, dtheta4/1, MATLAB Function/7(theta_dot_4)
  MATLAB Function/3(theta_ddot_3) -> ddtheta3/1, Integrator7/1
  Integrator8/1 -> theta3/1, MATLAB Function/2(theta_3)
  MATLAB Function/4(theta_ddot_4) -> Gain/1
  Saturation/1 -> Integrator5/1
  T2/1 -> MATLAB Function/9(T_2)
  T1/1 -> MATLAB Function/8(T_1)

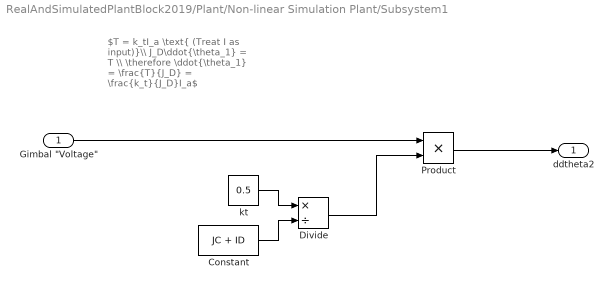
== system RealAndSimulatedPlantBlock2019/Plant/Non-linear Simulation Plant/Subsystem1 ==
  note: $T = k_tI_a \text{ (Treat I as input)}\\ J_D\ddot{\theta_1} = T \\ \therefore \ddot{\theta_1} = \frac{T}{J_D} = \frac{k_t}{J_D}I_a$
  "Gimbal \"Voltage\"" : Inport
  Constant : Constant  Value=JC + ID
  Divide : Product  Inputs=*/
  Product : Product
  kt : Constant  Value=0.5
  ddtheta2 : Outport
  wires:
  "Gimbal \"Voltage\""/1 -> Product/1
  kt/1 -> Divide/1
  Constant/1 -> Divide/2
  Product/1 -> ddtheta2/1
  Divide/1 -> Product/2

== system RealAndSimulatedPlantBlock2019/Plant/Non-linear Simulation Plant/ddtheta3 to force ==
  dtheta2 : Inport
  MATLAB Function : MATLAB Function  TreatAsAtomicUnit=on
  Force : Outport
  wires:
  MATLAB Function/1(F) -> Force/1
  dtheta2/1 -> MATLAB Function/1(dtheta2)

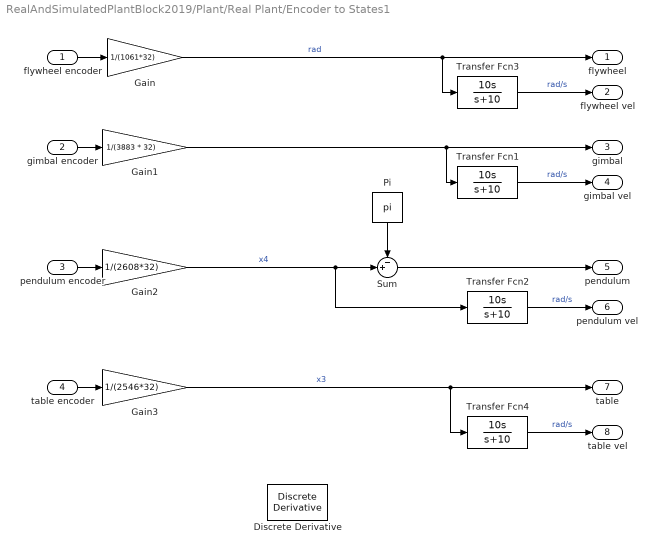
== system RealAndSimulatedPlantBlock2019/Plant/Real Plant/Encoder to States1 ==
  flywheel encoder : Inport
  gimbal encoder : Inport  Port=2
  pendulum encoder : Inport  Port=3
  table encoder : Inport  Port=4
  Discrete Derivative : simulink/Discrete/Discrete Derivative  gainval=1.0  ICPrevScaledInput=0.0  OutMin=[]  OutMax=[]  OutDataType=fixdt(1, 16)  OutScaling=2^-10  DoSatur=off
  Gain : Gain  Gain=1/(1061*32)
  Gain1 : Gain  Gain=1/(3883 * 32)
  Gain2 : Gain  Gain=1/(2608*32)
  Gain3 : Gain  Gain=1/(2546*32)
  Pi : Constant  Value=pi  OutDataTypeStr=Inherit: Inherit via back propagation
  Sum : Sum  Inputs=-+|
  Transfer Fcn{1..4} (4 alike) : TransferFcn  Numerator=[10 0 ]  Denominator=[1 10]
  flywheel : Outport
  flywheel vel : Outport  Port=2
  gimbal : Outport  Port=3
  gimbal vel : Outport  Port=4
  pendulum : Outport  Port=5
  pendulum vel : Outport  Port=6
  table : Outport  Port=7
  table vel : Outport  Port=8
  wires:
  flywheel encoder/1 -> Gain/1
  gimbal encoder/1 -> Gain1/1
  pendulum encoder/1 -> Gain2/1
  table encoder/1 -> Gain3/1
  Gain/1 -> Transfer Fcn3/1, flywheel/1  "rad"
  Transfer Fcn3/1 -> flywheel vel/1  "rad/s"
  Gain1/1 -> Transfer Fcn1/1, gimbal/1
  Transfer Fcn1/1 -> gimbal vel/1  "rad/s"
  Transfer Fcn2/1 -> pendulum vel/1  "rad/s"
  Gain3/1 -> Transfer Fcn4/1, table/1  "x3"
  Transfer Fcn4/1 -> table vel/1  "rad/s"
  Sum/1 -> pendulum/1
  Pi/1 -> Sum/1
  Gain2/1 -> Transfer Fcn2/1, Sum/2  "x4"

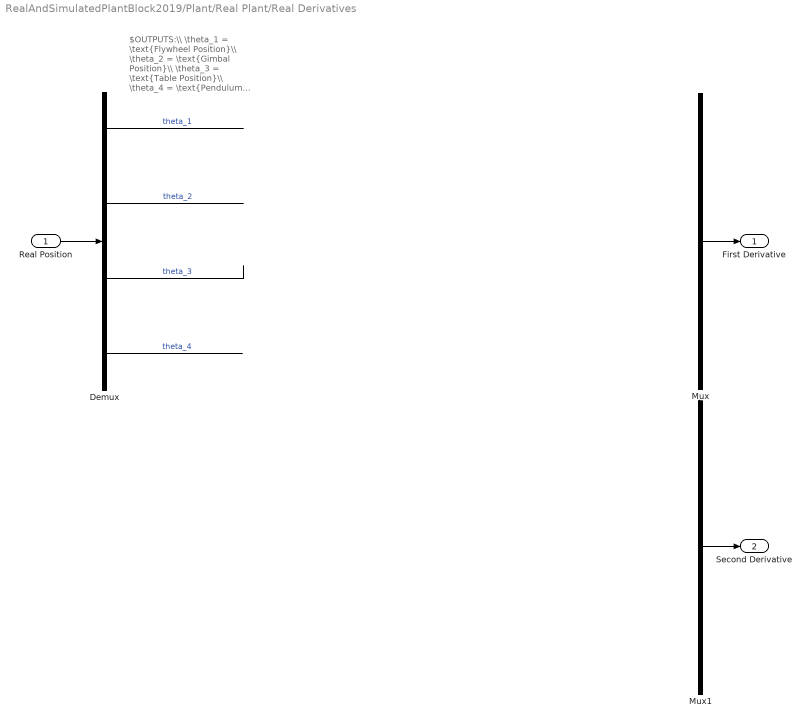
== system RealAndSimulatedPlantBlock2019/Plant/Real Plant/Real Derivatives ==
  note: $OUTPUTS:\\ \theta_1 = \text{Flywheel Position}\\ \theta_2 = \text{Gimbal Position}\\ \theta_3 = \text{Table Position}\\ \theta_4 = \text{Pendulum Position}\\$
  Real Position : Inport
  Demux : Demux
  Mux : Mux
  Mux1 : Mux
  First Derivative : Outport
  Second Derivative : Outport  Port=2
  wires:
  Real Position/1 -> Demux/1
  Demux/1 -> ?  "theta_1"
  Demux/2 -> ?  "theta_2"
  Demux/3 -> ?  "theta_3"
  Demux/4 -> ?  "theta_4"
  Mux/1 -> First Derivative/1
  Mux1/1 -> Second Derivative/1

== system RealAndSimulatedPlantBlock2019/Plant/Real Plant/Windows 10 ECPDSP Driver ==
  In1 : Inport
  S-Function : S-Function  FunctionName=ECPDSPDriver  Parameters=BaseAddr,STime,TimeOutPer,HWAccess  SFunctionDeploymentMode=off  EnableBusSupport=off
  Out1 : Outport
  wires:
  In1/1 -> S-Function/1
  S-Function/1 -> Out1/1

== matlab function RealAndSimulatedPlantBlock2019/Plant/Non-linear Simulation Plant/ddtheta3 to force/MATLAB Function ==
  data: dtheta2 input; F output
function F = fcn(dtheta2)
Jz_bar = 0.0131;
m = 0.1580;
l = 0.2698;
g = 9.81;
Rh = 0.37;
JD = 0.0273;
RotorSpeed=400; %RPM 
H=RotorSpeed*2*pi/60*JD;
T = H*dtheta2;
F = T/Rh;
